simulink model "part1_Signals"  (R2024a)
settings: Solver=VariableStepAuto  StartTime=0.0  StopTime=10.0  RelTol=1e-3
libraries: simulink_extras x1, dspsrcs4 x1, commrflib2 x1, spsTriangleGeneratorLib x1
settings Model: Creator=alice  LastModifiedBy=alice

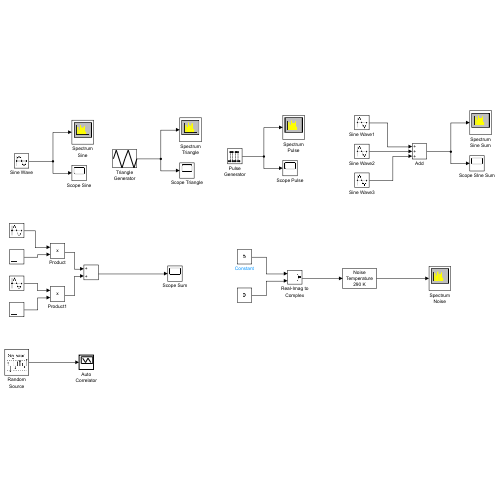
[thumbnail: Simulink's stored preview of the top-level diagram]
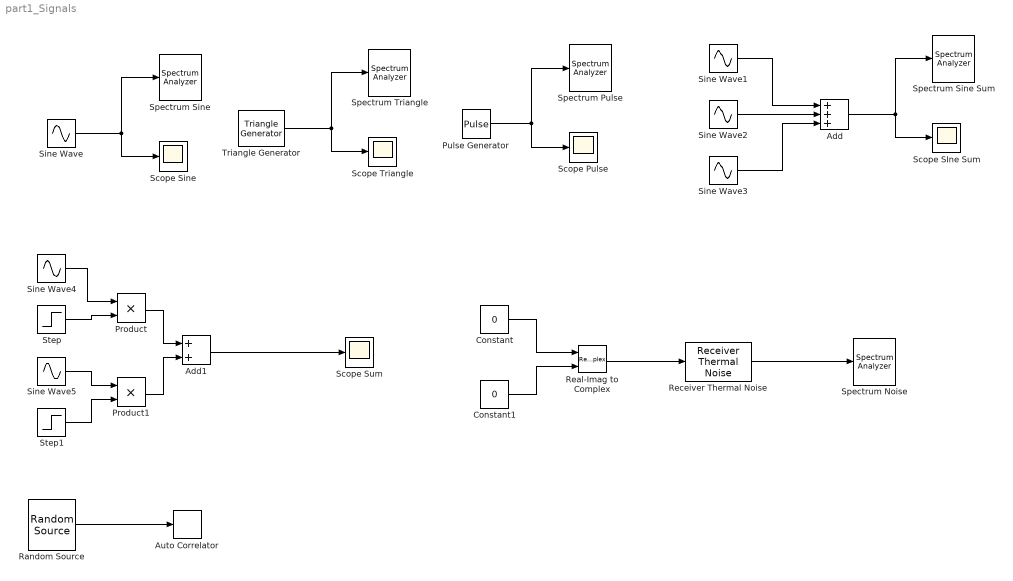
== system part1_Signals ==
  Add : Sum  Inputs=+++
  Add1 : Sum
  Auto Correlator : simulink_extras/Additional Sinks/Auto Correlator  npts=1024  HowOften=50  sampleT=1e-3
  Constant : Constant  Value=0  SampleTime=1e-6
  Constant1 : Constant  Value=0  SampleTime=1e-6
  Product : Product
  Product1 : Product
  Pulse Generator : DiscretePulseGenerator  Period=5000  PulseWidth=1000  SampleTime=1e-4
  Random Source : dspsrcs4/Random Source  SrcType=Gaussian  MinVal=0  MaxVal=1  MeanVal=0  VarVal=100  RepMode=Specify seed  rawSeed=1  IsInherit=off  SampTime=1e-3  SampFrame=1  OutComplex=Real  DataType=double  SimulateUsing=Interpreted execution
  Real-Imag to Complex : RealImagToComplex
  Receiver Thermal Noise : commrflib2/Receiver Thermal Noise  LegacyMode=off  NoiseMethod=Noise temperature  NoiseTemperature=290  NoiseFigure=3.0103  NoiseFactor=2  Add290KAntennaNoise=off  ReferenceLoad=1  RandomStream=Global stream  Seed=67987  SimulateUsing=Code generation
  Scope Pulse : Scope
  Scope SIne Sum : Scope
  Scope Sine : Scope
  Scope Sum : Scope
  Scope Triangle : Scope
  Sine Wave : Sin  SineType=Sample based  Amplitude=0.5  Samples=1000  SampleTime=1e-4
  Sine Wave1 : Sin  SineType=Sample based  Amplitude=0.5  Samples=1000  SampleTime=1e-4
  Sine Wave2 : Sin  SineType=Sample based  Amplitude=2  Samples=500  SampleTime=1e-4
  Sine Wave3 : Sin  SineType=Sample based  Amplitude=1.5  Samples=100  SampleTime=1e-4
  Sine Wave4 : Sin  SineType=Sample based  Amplitude=0.5  Samples=1000  SampleTime=1e-3
  Sine Wave5 : Sin  SineType=Sample based  Amplitude=0.5  Samples=1000  SampleTime=1e-3
  Spectrum Noise : SpectrumAnalyzer  WindowPosition=[0.000000,36.000000,1280.000000,521.000000,]  ScopeFrameLocation=window  Span=1000000  StartFrequency=-500000  StopFrequency=500000  YLimits=[-148.27653226,-140.9112126]  SelectedToolstripTab=spectrumAnalyzerToolstrip.channelMeasurementsTab
  Spectrum Pulse : SpectrumAnalyzer  WindowPosition=[0.000000,36.000000,1280.000000,521.000000,]  ScopeFrameLocation=window  Span=1000000  StartFrequency=-500000  StopFrequency=500000  YLimits=[-148.27653226,-140.9112126]  SelectedToolstripTab=spectrumAnalyzerToolstrip.channelMeasurementsTab
  Spectrum Sine : SpectrumAnalyzer  WindowPosition=[0.000000,36.000000,1280.000000,521.000000,]  ScopeFrameLocation=window  Span=1000000  StartFrequency=-500000  StopFrequency=500000  YLimits=[-148.27653226,-140.9112126]  SelectedToolstripTab=spectrumAnalyzerToolstrip.channelMeasurementsTab
  Spectrum Sine Sum : SpectrumAnalyzer  WindowPosition=[0.000000,36.000000,1280.000000,521.000000,]  ScopeFrameLocation=window  Span=1000000  StartFrequency=-500000  StopFrequency=500000  YLimits=[-148.27653226,-140.9112126]  SelectedToolstripTab=spectrumAnalyzerToolstrip.channelMeasurementsTab
  Spectrum Triangle : SpectrumAnalyzer  WindowPosition=[0.000000,36.000000,1280.000000,521.000000,]  ScopeFrameLocation=window  Span=1000000  StartFrequency=-500000  StopFrequency=500000  YLimits=[-148.27653226,-140.9112126]  SelectedToolstripTab=spectrumAnalyzerToolstrip.channelMeasurementsTab
  Step : Step  Time=2  SampleTime=0
  Step1 : Step  Time=4  SampleTime=0
  Triangle Generator : spsTriangleGeneratorLib/Triangle Generator  Freq=5  Phase=90  Ts=1e-4
  wires:
  Sine Wave1/1 -> Add/1
  Sine Wave2/1 -> Add/2
  Sine Wave3/1 -> Add/3
  Add1/1 -> Scope Sum/1
  Constant/1 -> Real-Imag to Complex/1
  Constant1/1 -> Real-Imag to Complex/2
  Real-Imag to Complex/1 -> Receiver Thermal Noise/1
  Random Source/1 -> Auto Correlator/1
  Sine Wave4/1 -> Product/1
  Step/1 -> Product/2
  Sine Wave5/1 -> Product1/1
  Step1/1 -> Product1/2
  Product/1 -> Add1/1
  Product1/1 -> Add1/2
  Add/1 -> Scope SIne Sum/1, Spectrum Sine Sum/1
  Receiver Thermal Noise/1 -> Spectrum Noise/1
  Sine Wave/1 -> Scope Sine/1, Spectrum Sine/1
  Triangle Generator/1 -> Scope Triangle/1, Spectrum Triangle/1
  Pulse Generator/1 -> Scope Pulse/1, Spectrum Pulse/1
